simulink model "Assignment1_V6"  (R2022b)
settings: Solver=FixedStepDiscrete  StartTime=0.0  StopTime=10.0  FixedStep=0.001  RelTol=1e-3  EnableMultiTasking=on
undefined symbols (not defined in the file or in its folder): A0, A1, D0, D1, D10, D11, D12, D13, D2, D3, D4, D5, D6, D7, D8, D9, PTA0, PTA1, PTA2, PTB2, PTB23, PTB3, PTB9, PTC16, PTC17, PTC2, PTC3, PTC4, PTD0, PTD1, PTD2, PTD3
libraries: frdmk64flib x19, simulink x4, etargetslib x2
settings Model: ExtModeTrigDuration=5  Creator=a laptop  LastModifiedBy=a laptop
settings SolverCC: AllowMultiTaskInputOutput=on  AutoInsertRateTranBlk=on  InsertRTBMode=Always
settings OptimizationCC: UseSpecifiedMinMax=on  StrengthReduction=on  PassReuseOutputArgsAs=Individual arguments  ZeroExternalMemoryAtStartup=off  ZeroInternalMemoryAtStartup=off  NoFixptDivByZeroProtection=on  EfficientFloat2IntCast=on  MaxStackSize=128  OptimizeBlockOrder=speed  OptimizationPriority=Speed  OptimizationCustomize=off  MultiThreadedLoops=on  EfficientTunableParamExpr=on
settings DebuggingCC: ParameterTunabilityLossMsg=error
settings HardwareCC: ProdBitPerPointer=32  ProdBitPerSizeT=32  ProdBitPerPtrDiffT=32  ProdLargestAtomicInteger=Long  ProdLargestAtomicFloat=Double  ProdWordSize=32  ProdLongLongMode=on  ProdHWDeviceType=ARM Compatible->ARM Cortex
settings SFSimCC: MATLABDynamicMemAlloc=off
settings RTWCC: Description=Embedded Coder  SystemTargetFile=ert.tlc  HardwareBoard=NXP FRDM-K64F  TLCOptions="-aInlineSetEventsForThisBaseRateFcn=TLC_FALSE -aSuppressMultiTaskScheduler=TLC_FALSE  -aRateBasedStepFcn=0"  TemplateMakefile=ert_default_tmf  Toolchain=GNU Tools for ARM Embedded Processors  BuildConfiguration=Faster Runs
settings CodeAppCC: ForceParamTrailComments=on  IgnoreCustomStorageClasses=off  OperatorAnnotations=on  SimulinkDataObjDesc=on  SFDataObjDesc=on  InsertBlockDesc=on
settings ERTTargetCC: SupportNonFinite=off  SupportComplex=off  SupportVariableSizeSignals=on  ExtModeTransport=4  ExtModeMexFile=sendToCommService

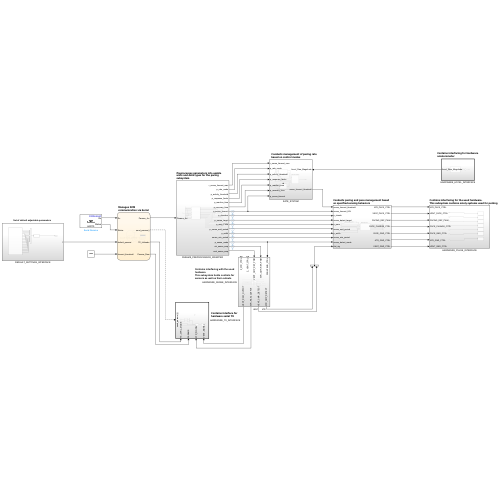
[thumbnail: Simulink's stored preview of the top-level diagram]
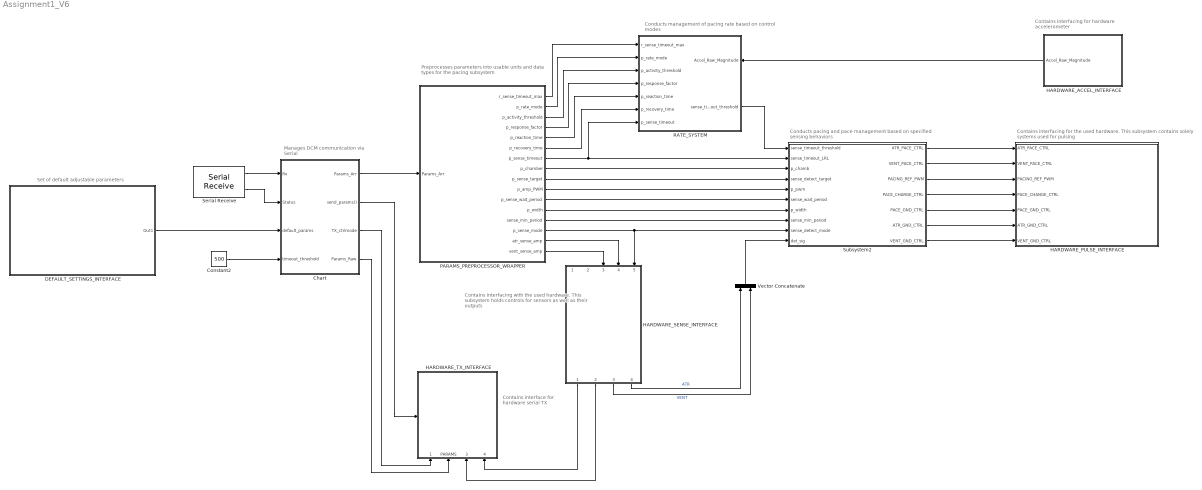
== system Assignment1_V6 ==
  note: Manages DCM communication via Serial
  note: Contains interface for hardware serial TX
  note: Contains interfacing for hardware accelerometer
  note: Conducts management of pacing rate based on control modes
  note: Set of default adjustable parameters
  note: Conducts pacing and pace management based on specified sensing behaviors
  note: Preprocesses parameters into usable units and data types for the pacing subsystem
  note: Contains interfacing for the used hardware.
      | This subsystem contains solely systems used for pulsing
  note: Contains interfacing with the used hardware.
      | This subsystem holds controls for sensors as well as their outputs
  Chart : Stateflow chart  TreatAsAtomicUnit=on
      settings: PortSchema="{\"entries\":[{\"content\":{\"sides\":[{\"content\":{\"connectorIds\":[\"In1\",\"In2\",\"In3\",\"In4\"]},\"type\":\"ConnectorPlacement.EquallySpacedRectSide\",\"uuid\":\"320bc760-8283-4f2b-996b-2bacb632d8d9\"},{\"content\":{\"connectorIds\":[\"Out2\",\"Out4\",\"Out3\",\"Out1\"],\"side\":\"RIGHT\"},\"type\":\"ConnectorPlacement.EquallySpacedRectSide\",\"uuid\":\"405a4bb2-50d6-4c0d-b540-a004b1136e76\"},{\"content\":{\"connectorIds\":[],\"side\":\"TOP\"},\"type\":\"ConnectorPlacement.EquallySpacedRectSide\",\"uuid\":\"abc74140-9996-448b-8aab-969529bb67e5\"}]},\"type\":\"ConnectorPlacement.EquallySpacedConnector\",\"uuid\":\"83b64870-f027-44a6-ac9f-b34b790ab38f\"}],\"packageUris\":[\"http://schema.mathworks.com/mf0/Connector/R2020b\"],\"version\":\"1.0\"}"
  Constant2 : Constant  Value=500
  DEFAULT_SETTINGS_INTERFACE : Subsystem
  HARDWARE_ACCEL_INTERFACE : Subsystem  TreatAsAtomicUnit=on
  HARDWARE_PULSE_INTERFACE : Subsystem
  HARDWARE_SENSE_INTERFACE : Subsystem
  HARDWARE_TX_INTERFACE : Subsystem
  PARAMS_PREPROCESSOR_WRAPPER : Subsystem
  RATE_SYSTEM : Subsystem
      settings: PortSchema="{\"entries\":[{\"content\":{\"sides\":[{\"content\":{\"connectorIds\":[\"In1\",\"In2\",\"In3\",\"In4\",\"In5\",\"In6\",\"In7\"]},\"type\":\"ConnectorPlacement.EquallySpacedRectSide\",\"uuid\":\"da911c89-d0b6-46c9-8ca4-48906cb25f38\"},{\"content\":{\"connectorIds\":[\"In8\",\"Out1\"],\"side\":\"RIGHT\"},\"type\":\"ConnectorPlacement.EquallySpacedRectSide\",\"uuid\":\"d13d5404-7ff7-47d0-a9a2-e0a3ff932734\"},{\"content\":{\"connectorIds\":[],\"side\":\"TOP\"},\"type\":\"ConnectorPlacement.EquallySpacedRectSide\",\"uuid\":\"daee8f81-06de-4c9b-88e4-466b0c826808\"}]},\"type\":\"ConnectorPlacement.EquallySpacedConnector\",\"uuid\":\"a6134fa8-7280-4bb4-a6f1-cb05dfad6031\"}],\"packageUris\":[\"http://schema.mathworks.com/mf0/Connector/R2020b\"],\"version\":\"1.0\"}"
  Serial Receive : frdmk64flib/Serial Receive  SCIModule=0  Baudrate=uint32(9600)  Parity=None  StopBits=1  HardwareFlowControl=None  ByteOrder=LittleEndian  DataType=uint8  DataLength=16  BlockingMode=off  OutputStatus=on  SampleTime=-1
  Subsystem2 : Subsystem
  Vector Concatenate : Concatenate
  wires:
  Serial Receive/1 -> Chart/1(Rx)
  HARDWARE_SENSE_INTERFACE/4(ATR_CMP_DETECT) -> Vector Concatenate/1  "ATR"
  Constant2/1 -> Chart/4(timeout_threshold)
  HARDWARE_SENSE_INTERFACE/3(VENT_CMP_DETECT) -> Vector Concatenate/2  "VENT"
  PARAMS_PREPROCESSOR_WRAPPER/1(r_sense_timeout_max) -> RATE_SYSTEM/1(r_sense_timeout_max)
  HARDWARE_SENSE_INTERFACE/2(ATR_RAW_OUTPUT) -> HARDWARE_TX_INTERFACE/3(ATR_SIGNAL)
  Serial Receive/2 -> Chart/2(Status)
  PARAMS_PREPROCESSOR_WRAPPER/5(p_reaction_time) -> RATE_SYSTEM/5(p_reaction_time)
  Chart/3(TX_ctrlmode) -> HARDWARE_TX_INTERFACE/1(TX_CTRL_MODE)
  PARAMS_PREPROCESSOR_WRAPPER/6(p_recovery_time) -> RATE_SYSTEM/6(p_recovery_time)
  PARAMS_PREPROCESSOR_WRAPPER/14(p_sense_mode) -> Subsystem2/9(sense_detect_mode), HARDWARE_SENSE_INTERFACE/5(FRONTEND_CTRL)
  PARAMS_PREPROCESSOR_WRAPPER/2(p_rate_mode) -> RATE_SYSTEM/2(p_rate_mode)
  PARAMS_PREPROCESSOR_WRAPPER/4(p_response_factor) -> RATE_SYSTEM/4(p_response_factor)
  Chart/1(Params_Raw) -> HARDWARE_TX_INTERFACE/2(PARAMS)
  PARAMS_PREPROCESSOR_WRAPPER/16(vent_sense_amp) -> HARDWARE_SENSE_INTERFACE/3(VENT_CMP_REF_PWM)
  PARAMS_PREPROCESSOR_WRAPPER/3(p_activity_threshold) -> RATE_SYSTEM/3(p_activity_threshold)
  HARDWARE_SENSE_INTERFACE/1(VENT_RAW_OUTPUT) -> HARDWARE_TX_INTERFACE/4(VENT_SIGNAL)
  PARAMS_PREPROCESSOR_WRAPPER/15(atr_sense_amp) -> HARDWARE_SENSE_INTERFACE/4(ATR_CMP_REF_PWM)
  HARDWARE_ACCEL_INTERFACE/1(Accel_Raw_Magnitude) -> RATE_SYSTEM/8(Accel_Raw_Magnitude)
  PARAMS_PREPROCESSOR_WRAPPER/7(p_sense_timeout) -> Subsystem2/2(sense_timeout_LRL), RATE_SYSTEM/7(p_sense_timeout)
  Chart/2(Params_Arr) -> PARAMS_PREPROCESSOR_WRAPPER/1(Params_Arr)
  Chart/4(send_params()) -> HARDWARE_TX_INTERFACE/Trigger
  PARAMS_PREPROCESSOR_WRAPPER/8(p_chamber) -> Subsystem2/3(p_chamb)
  PARAMS_PREPROCESSOR_WRAPPER/9(p_sense_target) -> Subsystem2/4(sense_detect_target)
  RATE_SYSTEM/1(sense_timeout_threshold) -> Subsystem2/1(sense_timeout_threshold)
  PARAMS_PREPROCESSOR_WRAPPER/10(p_amp_PWM) -> Subsystem2/5(p_pwm)
  PARAMS_PREPROCESSOR_WRAPPER/11(p_sense_wait_period) -> Subsystem2/6(sense_wait_period)
  PARAMS_PREPROCESSOR_WRAPPER/12(p_width) -> Subsystem2/7(p_width)
  Vector Concatenate/1 -> Subsystem2/10(det_sig)
  PARAMS_PREPROCESSOR_WRAPPER/13(sense_min_period) -> Subsystem2/8(sense_min_period)
  Subsystem2/1(ATR_PACE_CTRL) -> HARDWARE_PULSE_INTERFACE/1(ATR_PACE_CTRL)
  Subsystem2/2(VENT_PACE_CTRL) -> HARDWARE_PULSE_INTERFACE/2(VENT_PACE_CTRL)
  Subsystem2/3(PACING_REF_PWM) -> HARDWARE_PULSE_INTERFACE/3(PACING_REF_PWM)
  Subsystem2/4(PACE_CHARGE_CTRL) -> HARDWARE_PULSE_INTERFACE/4(PACE_CHANGE_CTRL)
  Subsystem2/5(PACE_GND_CTRL) -> HARDWARE_PULSE_INTERFACE/5(PACE_GND_CTRL)
  Subsystem2/6(ATR_GND_CTRL) -> HARDWARE_PULSE_INTERFACE/6(ATR_GND_CTRL)
  Subsystem2/7(VENT_GND_CTRL) -> HARDWARE_PULSE_INTERFACE/7(VENT_GND_CTRL)
  DEFAULT_SETTINGS_INTERFACE/1(Out1) -> Chart/3(default_params)

== system Assignment1_V6/DEFAULT_SETTINGS_INTERFACE ==
  Cast : DataTypeConversion  OutDataTypeStr=uint8  SaturateOnIntegerOverflow=off  RndMeth=Floor
  DEFAULT_PARAMS : Subsystem
  Vector Concatenate1 : Concatenate  NumInputs=15
  Out1 : Outport
  wires:
  DEFAULT_PARAMS/15(RECOVERY_TIME) -> Vector Concatenate1/15
  DEFAULT_PARAMS/9(VENT_PULSE_WIDTH) -> Vector Concatenate1/9
  DEFAULT_PARAMS/3(UPPER_RATE_LIMIT) -> Vector Concatenate1/3
  Vector Concatenate1/1 -> Cast/1
  DEFAULT_PARAMS/4(MAXIMUM_SENSOR_RATE) -> Vector Concatenate1/4
  DEFAULT_PARAMS/14(RESPONSE_FAC) -> Vector Concatenate1/14
  DEFAULT_PARAMS/7(ATR_SENSE_THRESHOLD) -> Vector Concatenate1/7
  DEFAULT_PARAMS/6(ATR_PULSE_WIDTH) -> Vector Concatenate1/6
  DEFAULT_PARAMS/1(PACE_MODE) -> Vector Concatenate1/1
  DEFAULT_PARAMS/8(VENT_PUL_AMPLITUDE) -> Vector Concatenate1/8
  DEFAULT_PARAMS/12(VENT_REFRACTORY_PERIOD) -> Vector Concatenate1/12
  DEFAULT_PARAMS/10(VENT_SENSE_THRESHOLD) -> Vector Concatenate1/10
  DEFAULT_PARAMS/13(REACTION_TIME) -> Vector Concatenate1/13
  DEFAULT_PARAMS/5(ATR_PUL_AMPLITUDE) -> Vector Concatenate1/5
  DEFAULT_PARAMS/2(LOWER_RATE_LIMIT) -> Vector Concatenate1/2
  DEFAULT_PARAMS/11(ATR_REFRACTORY_PERIOD) -> Vector Concatenate1/11
  Cast/1 -> Out1/1

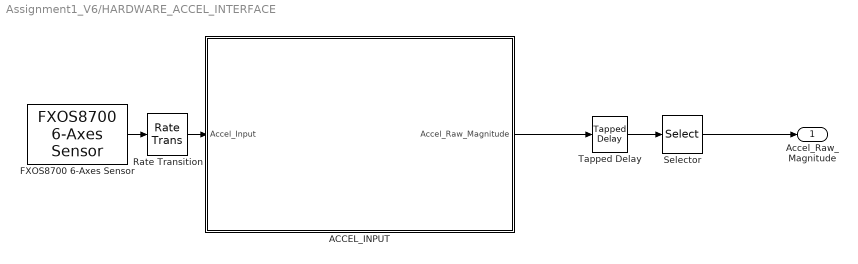
== system Assignment1_V6/HARDWARE_ACCEL_INTERFACE ==
  ACCEL_INPUT : Subsystem
  FXOS8700 6-Axes Sensor : frdmk64flib/FXOS8700 6-Axes Sensor  Activesensor=Accelerometer only  ODR=800Hz  HybridODR=400Hz  Accelfullrange=-4g to +4g  SampleTime=-1
  Rate Transition : RateTransition  Deterministic=off  OutPortSampleTime=0.002
  Selector : Selector  InputPortWidth=50  IndexOptions=Index vector (dialog)  Indices=1  OutputSizes=1
  Tapped Delay : simulink/Discrete/Tapped Delay  vinit=0.0  samptime=0.002  NumDelays=49  DelayOrder=Oldest  includeCurrent=on
  Accel_Raw_Magnitude : Outport
  wires:
  FXOS8700 6-Axes Sensor/1 -> Rate Transition/1
  Tapped Delay/1 -> Selector/1
  Selector/1 -> Accel_Raw_Magnitude/1
  ACCEL_INPUT/1(Accel_Raw_Magnitude) -> Tapped Delay/1
  Rate Transition/1 -> ACCEL_INPUT/1(Accel_Input)

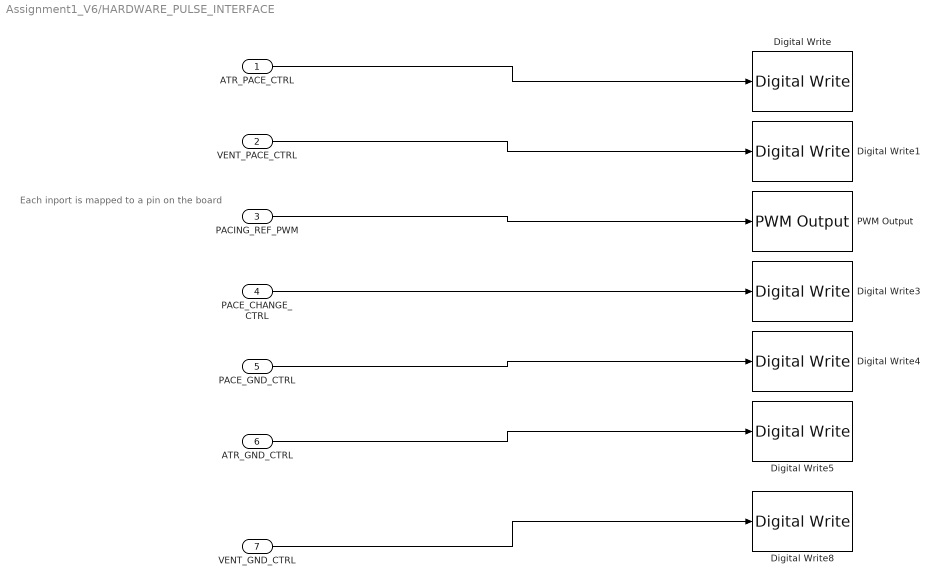
== system Assignment1_V6/HARDWARE_PULSE_INTERFACE ==
  note: Each inport is mapped to a pin on the board
  ATR_PACE_CTRL : Inport
  VENT_PACE_CTRL : Inport  Port=2
  PACING_REF_PWM : Inport  Port=3
  PACE_CHANGE_CTRL : Inport  Port=4
  PACE_GND_CTRL : Inport  Port=5
  ATR_GND_CTRL : Inport  Port=6
  VENT_GND_CTRL : Inport  Port=7
  Digital Write : frdmk64flib/Digital Write  Whichpin=PTA0 (D8)
  Digital Write1 : frdmk64flib/Digital Write  Whichpin=PTC4 (D9)
  Digital Write3 : frdmk64flib/Digital Write  Whichpin=PTB9 (D2)
  Digital Write4 : frdmk64flib/Digital Write  Whichpin=PTD0 (D10)
  Digital Write5 : frdmk64flib/Digital Write  Whichpin=PTD2 (D11)
  Digital Write8 : frdmk64flib/Digital Write  Whichpin=PTD3 (D12)
  PWM Output : frdmk64flib/PWM Output  Whichpin=PTA2 (D5)  InitialFrequency=2000  InitialDutyCycle=0
  wires:
  PACE_CHANGE_CTRL/1 -> Digital Write3/1
  PACE_GND_CTRL/1 -> Digital Write4/1
  VENT_PACE_CTRL/1 -> Digital Write1/1
  VENT_GND_CTRL/1 -> Digital Write8/1
  ATR_PACE_CTRL/1 -> Digital Write/1
  ATR_GND_CTRL/1 -> Digital Write5/1
  PACING_REF_PWM/1 -> PWM Output/1

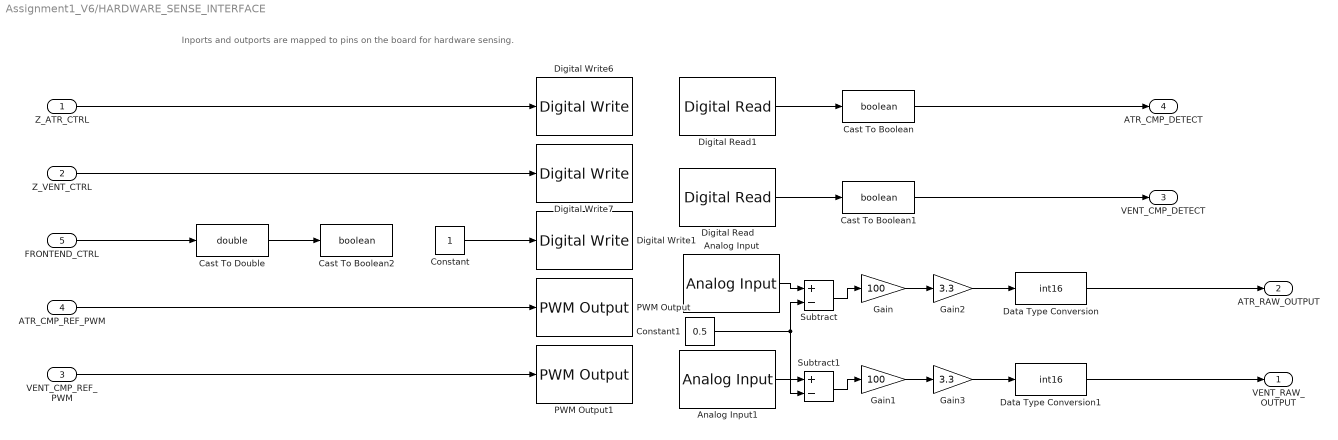
== system Assignment1_V6/HARDWARE_SENSE_INTERFACE ==
  note: Inports and outports are mapped to pins on the board for hardware sensing.
  Z_ATR_CTRL : Inport
  Z_VENT_CTRL : Inport  Port=2
  VENT_CMP_REF_PWM : Inport  Port=3
  ATR_CMP_REF_PWM : Inport  Port=4
  FRONTEND_CTRL : Inport  Port=5
  Analog Input : frdmk64flib/Analog Input  Whichpin=PTB2 (A0)  SampleTime=-1
  Analog Input1 : frdmk64flib/Analog Input  Whichpin=PTB3 (A1)  SampleTime=-1
  Cast To Boolean : DataTypeConversion  OutDataTypeStr=boolean  RndMeth=Round  SaturateOnIntegerOverflow=off
  Cast To Boolean1 : DataTypeConversion  OutDataTypeStr=boolean  RndMeth=Round  SaturateOnIntegerOverflow=off
  Cast To Boolean2 : DataTypeConversion  OutDataTypeStr=boolean  SaturateOnIntegerOverflow=off  RndMeth=Floor
  Cast To Double : DataTypeConversion  OutDataTypeStr=double  SaturateOnIntegerOverflow=off  RndMeth=Floor
  Constant : Constant
  Constant1 : Constant  Value=0.5
  Data Type Conversion : DataTypeConversion  OutDataTypeStr=int16  RndMeth=Nearest  SaturateOnIntegerOverflow=off
  Data Type Conversion1 : DataTypeConversion  OutDataTypeStr=int16  RndMeth=Nearest  SaturateOnIntegerOverflow=off
  Digital Read : frdmk64flib/Digital Read  Whichpin=PTC17 (D1)  SampleTime=-1
  Digital Read1 : frdmk64flib/Digital Read  Whichpin=PTC16 (D0)  SampleTime=-1
  Digital Write1 : frdmk64flib/Digital Write  Whichpin=PTD1 (D13)
  Digital Write6 : frdmk64flib/Digital Write  Whichpin=PTB23 (D4)
  Digital Write7 : frdmk64flib/Digital Write  Whichpin=PTC3 (D7)
  Gain : Gain  Gain=100
  Gain1 : Gain  Gain=100
  Gain2 : Gain  Gain=3.3
  Gain3 : Gain  Gain=3.3
  PWM Output : frdmk64flib/PWM Output  Whichpin=PTC2 (D6)  InitialFrequency=2000  InitialDutyCycle=0
  PWM Output1 : frdmk64flib/PWM Output  Whichpin=PTA1 (D3)  InitialFrequency=2000  InitialDutyCycle=0
  Subtract : Sum  Inputs=+-
  Subtract1 : Sum  Inputs=+-
  VENT_RAW_OUTPUT : Outport
  ATR_RAW_OUTPUT : Outport  Port=2
  VENT_CMP_DETECT : Outport  Port=3
  ATR_CMP_DETECT : Outport  Port=4  OutDataTypeStr=boolean
  wires:
  Z_ATR_CTRL/1 -> Digital Write6/1
  Z_VENT_CTRL/1 -> Digital Write7/1
  FRONTEND_CTRL/1 -> Cast To Double/1
  ATR_CMP_REF_PWM/1 -> PWM Output/1
  VENT_CMP_REF_PWM/1 -> PWM Output1/1
  Digital Read1/1 -> Cast To Boolean/1
  Digital Read/1 -> Cast To Boolean1/1
  Cast To Double/1 -> Cast To Boolean2/1
  Gain/1 -> Gain2/1
  Gain1/1 -> Gain3/1
  Data Type Conversion/1 -> ATR_RAW_OUTPUT/1
  Data Type Conversion1/1 -> VENT_RAW_OUTPUT/1
  Gain2/1 -> Data Type Conversion/1
  Gain3/1 -> Data Type Conversion1/1
  Constant/1 -> Digital Write1/1
  Analog Input/1 -> Subtract/1
  Subtract/1 -> Gain/1
  Analog Input1/1 -> Subtract1/1
  Subtract1/1 -> Gain1/1
  Constant1/1 -> Subtract1/2, Subtract/2
  Cast To Boolean/1 -> ATR_CMP_DETECT/1
  Cast To Boolean1/1 -> VENT_CMP_DETECT/1

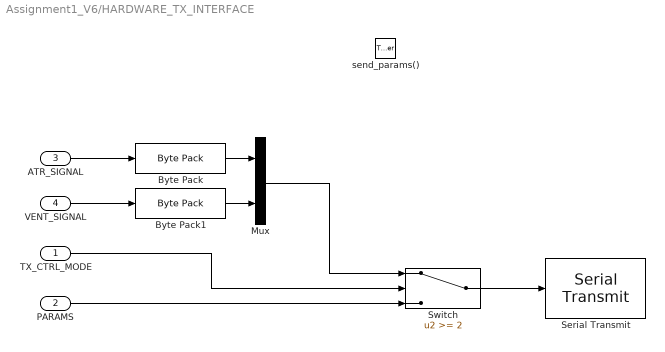
== system Assignment1_V6/HARDWARE_TX_INTERFACE ==
  TX_CTRL_MODE : Inport
  PARAMS : Inport  Port=2  OutDataTypeStr=uint8
  ATR_SIGNAL : Inport  Port=3
  VENT_SIGNAL : Inport  Port=4
  send_params() : TriggerPort  TriggerType=function-call  FunctionName=send_params  VariantControl=(inherit)
  Byte Pack : etargetslib/Byte Pack  datatypes={'int16'}  byteAlign=1
  Byte Pack1 : etargetslib/Byte Pack  datatypes={'int16'}  byteAlign=1
  Mux : Mux  Inputs=2
  Serial Transmit : frdmk64flib/Serial Transmit  SCIModule=0  Baudrate=uint32(9600)  Parity=None  StopBits=1  HardwareFlowControl=None  ByteOrder=LittleEndian  BlockingMode=on  OutputStatus=off
  Switch : Switch  Threshold=2  OutDataTypeStr=uint8  SaturateOnIntegerOverflow=off  InputSameDT=off
  wires:
  Byte Pack1/1 -> Mux/2
  Byte Pack/1 -> Mux/1
  ATR_SIGNAL/1 -> Byte Pack/1
  VENT_SIGNAL/1 -> Byte Pack1/1
  Switch/1 -> Serial Transmit/1
  Mux/1 -> Switch/1
  TX_CTRL_MODE/1 -> Switch/2
  PARAMS/1 -> Switch/3

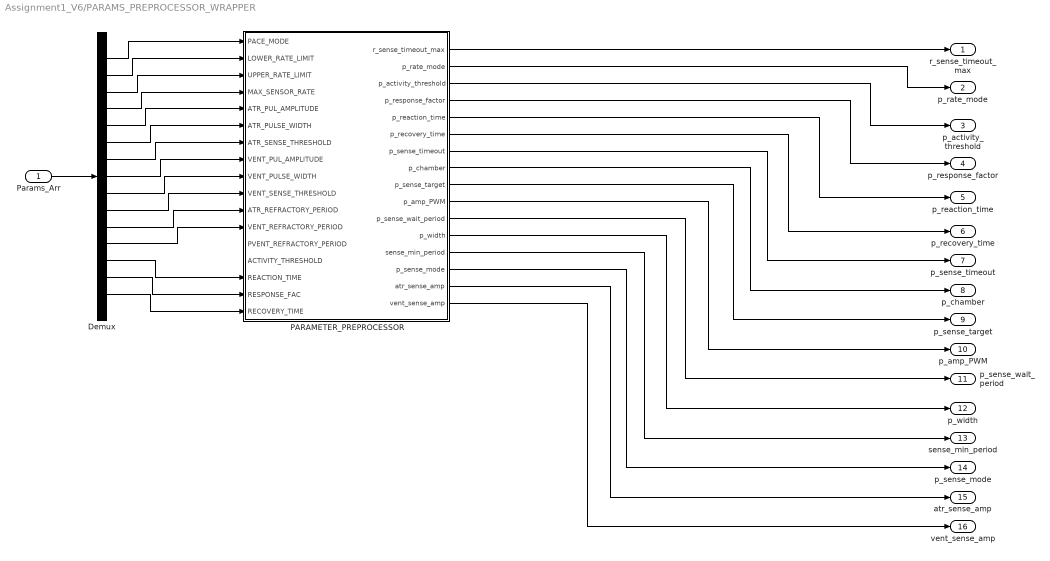
== system Assignment1_V6/PARAMS_PREPROCESSOR_WRAPPER ==
  Params_Arr : Inport
  Demux : Demux  Outputs=15
  PARAMETER_PREPROCESSOR : Subsystem
  r_sense_timeout_max : Outport
  p_rate_mode : Outport  Port=2
  p_activity_threshold : Outport  Port=3
  p_response_factor : Outport  Port=4
  p_reaction_time : Outport  Port=5
  p_recovery_time : Outport  Port=6
  p_sense_timeout : Outport  Port=7
  p_chamber : Outport  Port=8
  p_sense_target : Outport  Port=9
  p_amp_PWM : Outport  Port=10
  p_sense_wait_period : Outport  Port=11
  p_width : Outport  Port=12
  sense_min_period : Outport  Port=13
  p_sense_mode : Outport  Port=14
  atr_sense_amp : Outport  Port=15
  vent_sense_amp : Outport  Port=16
  wires:
  PARAMETER_PREPROCESSOR/11(p_sense_wait_period) -> p_sense_wait_period/1
  PARAMETER_PREPROCESSOR/9(p_sense_target) -> p_sense_target/1
  PARAMETER_PREPROCESSOR/8(p_chamber) -> p_chamber/1
  PARAMETER_PREPROCESSOR/3(p_activity_threshold) -> p_activity_threshold/1
  PARAMETER_PREPROCESSOR/16(vent_sense_amp) -> vent_sense_amp/1
  PARAMETER_PREPROCESSOR/12(p_width) -> p_width/1
  PARAMETER_PREPROCESSOR/15(atr_sense_amp) -> atr_sense_amp/1
  PARAMETER_PREPROCESSOR/14(p_sense_mode) -> p_sense_mode/1
  PARAMETER_PREPROCESSOR/5(p_reaction_time) -> p_reaction_time/1
  PARAMETER_PREPROCESSOR/10(p_amp_PWM) -> p_amp_PWM/1
  PARAMETER_PREPROCESSOR/13(sense_min_period) -> sense_min_period/1
  PARAMETER_PREPROCESSOR/1(r_sense_timeout_max) -> r_sense_timeout_max/1
  PARAMETER_PREPROCESSOR/4(p_response_factor) -> p_response_factor/1
  PARAMETER_PREPROCESSOR/2(p_rate_mode) -> p_rate_mode/1
  PARAMETER_PREPROCESSOR/7(p_sense_timeout) -> p_sense_timeout/1
  PARAMETER_PREPROCESSOR/6(p_recovery_time) -> p_recovery_time/1
  Params_Arr/1 -> Demux/1
  Demux/15 -> PARAMETER_PREPROCESSOR/17(RECOVERY_TIME)
  Demux/14 -> PARAMETER_PREPROCESSOR/16(RESPONSE_FAC)
  Demux/13 -> PARAMETER_PREPROCESSOR/15(REACTION_TIME)
  Demux/12 -> PARAMETER_PREPROCESSOR/12(VENT_REFRACTORY_PERIOD)
  Demux/11 -> PARAMETER_PREPROCESSOR/11(ATR_REFRACTORY_PERIOD)
  Demux/10 -> PARAMETER_PREPROCESSOR/10(VENT_SENSE_THRESHOLD)
  Demux/9 -> PARAMETER_PREPROCESSOR/9(VENT_PULSE_WIDTH)
  Demux/8 -> PARAMETER_PREPROCESSOR/8(VENT_PUL_AMPLITUDE)
  Demux/7 -> PARAMETER_PREPROCESSOR/7(ATR_SENSE_THRESHOLD)
  Demux/6 -> PARAMETER_PREPROCESSOR/6(ATR_PULSE_WIDTH)
  Demux/5 -> PARAMETER_PREPROCESSOR/5(ATR_PUL_AMPLITUDE)
  Demux/4 -> PARAMETER_PREPROCESSOR/4(MAX_SENSOR_RATE)
  Demux/3 -> PARAMETER_PREPROCESSOR/3(UPPER_RATE_LIMIT)
  Demux/2 -> PARAMETER_PREPROCESSOR/2(LOWER_RATE_LIMIT)
  Demux/1 -> PARAMETER_PREPROCESSOR/1(PACE_MODE)

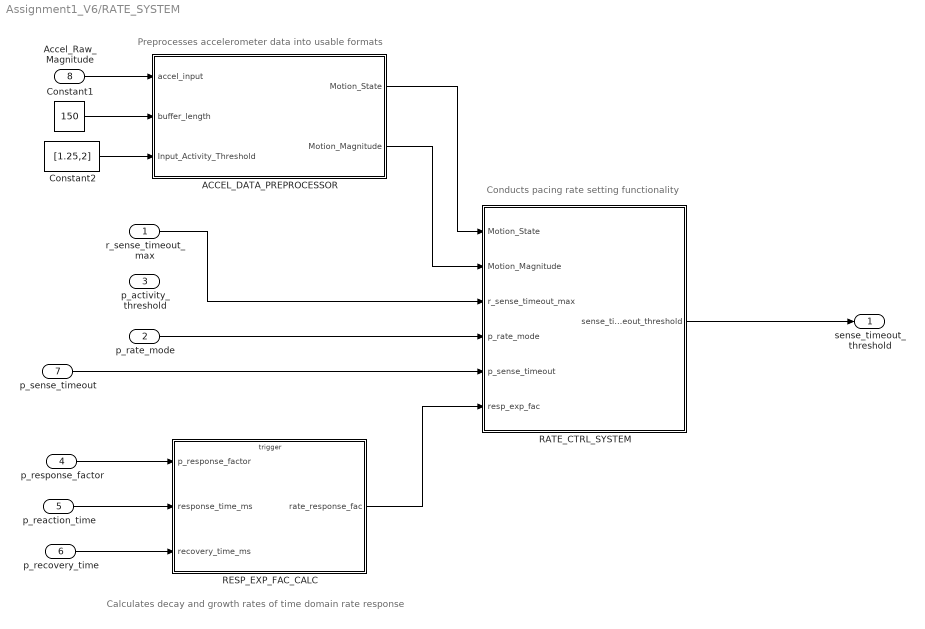
== system Assignment1_V6/RATE_SYSTEM ==
  note: Preprocesses accelerometer data into usable formats
  note: Calculates decay and growth rates of time domain rate response
  note: Conducts pacing rate setting functionality
  r_sense_timeout_max : Inport
  p_rate_mode : Inport  Port=2
  p_activity_threshold : Inport  Port=3
  p_response_factor : Inport  Port=4
  p_reaction_time : Inport  Port=5
  p_recovery_time : Inport  Port=6
  p_sense_timeout : Inport  Port=7
  Accel_Raw_Magnitude : Inport  Port=8
  ACCEL_DATA_PREPROCESSOR : Subsystem
  Constant1 : Constant  Value=150
  Constant2 : Constant  Value=[1.25,2]
  RATE_CTRL_SYSTEM : Stateflow chart  TreatAsAtomicUnit=on
  RESP_EXP_FAC_CALC : Subsystem
  sense_timeout_threshold : Outport
  wires:
  p_rate_mode/1 -> RATE_CTRL_SYSTEM/4(p_rate_mode)
  r_sense_timeout_max/1 -> RATE_CTRL_SYSTEM/3(r_sense_timeout_max)
  p_sense_timeout/1 -> RATE_CTRL_SYSTEM/5(p_sense_timeout)
  Constant2/1 -> ACCEL_DATA_PREPROCESSOR/3(Input_Activity_Threshold)
  Constant1/1 -> ACCEL_DATA_PREPROCESSOR/2(buffer_length)
  Accel_Raw_Magnitude/1 -> ACCEL_DATA_PREPROCESSOR/1(accel_input)
  RATE_CTRL_SYSTEM/1(sense_timeout_threshold) -> sense_timeout_threshold/1
  ACCEL_DATA_PREPROCESSOR/2(Motion_Magnitude) -> RATE_CTRL_SYSTEM/2(Motion_Magnitude)
  ACCEL_DATA_PREPROCESSOR/1(Motion_State) -> RATE_CTRL_SYSTEM/1(Motion_State)
  p_response_factor/1 -> RESP_EXP_FAC_CALC/1(p_response_factor)
  p_reaction_time/1 -> RESP_EXP_FAC_CALC/2(response_time_ms)
  p_recovery_time/1 -> RESP_EXP_FAC_CALC/3(recovery_time_ms)
  RESP_EXP_FAC_CALC/1(rate_response_fac) -> RATE_CTRL_SYSTEM/6(resp_exp_fac)

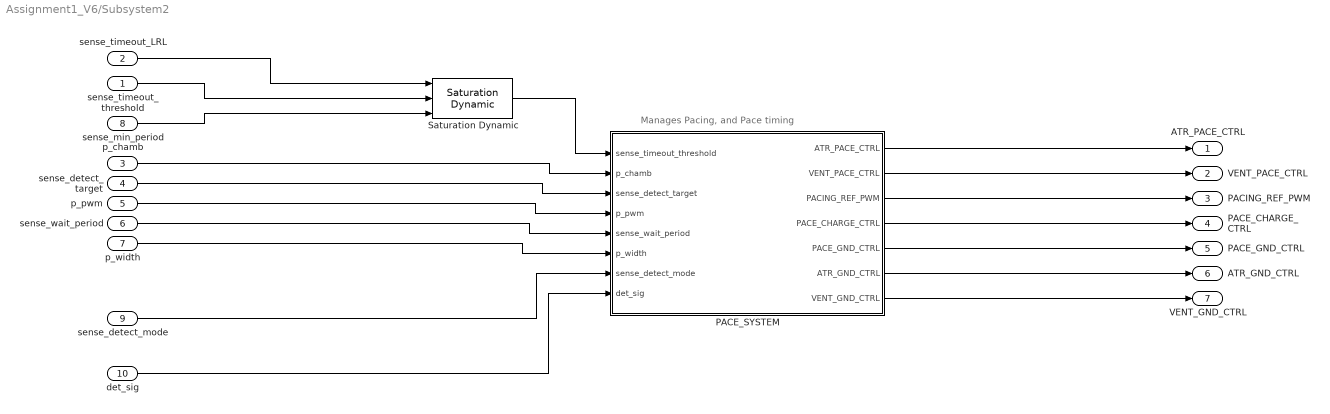
== system Assignment1_V6/Subsystem2 ==
  note: Manages Pacing, and Pace timing
  sense_timeout_threshold : Inport
  sense_timeout_LRL : Inport  Port=2
  p_chamb : Inport  Port=3
  sense_detect_target : Inport  Port=4
  p_pwm : Inport  Port=5
  sense_wait_period : Inport  Port=6
  p_width : Inport  Port=7
  sense_min_period : Inport  Port=8
  sense_detect_mode : Inport  Port=9
  det_sig : Inport  Port=10
  PACE_SYSTEM : Stateflow chart  TreatAsAtomicUnit=on
      settings: PortSchema="{\"entries\":[{\"content\":{\"sides\":[{\"content\":{\"connectorIds\":[\"In3\",\"In1\",\"In2\",\"In4\",\"In5\",\"In6\",\"In7\",\"In8\"]},\"type\":\"ConnectorPlacement.EquallySpacedRectSide\",\"uuid\":\"7443a3c3-e653-4ca7-8541-eabcfaf454bc\"},{\"content\":{\"connectorIds\":[\"Out1\",\"Out2\",\"Out3\",\"Out4\",\"Out5\",\"Out6\",\"Out7\"],\"side\":\"RIGHT\"},\"type\":\"ConnectorPlacement.EquallySpacedRectSide\",\"uuid\":\"2c63cfa0-dfd9-4a62-91aa-a60ecd75cc2c\"},{\"content\":{\"connectorIds\":[],\"side\":\"TOP\"},\"type\":\"ConnectorPlacement.EquallySpacedRectSide\",\"uuid\":\"5c2dbe0e-7e89-449d-bdd0-c0f7e700edae\"}]},\"type\":\"ConnectorPlacement.EquallySpacedConnector\",\"uuid\":\"602c7a1c-8730-4b31-b945-266bd0371e8b\"}],\"packageUris\":[\"http://schema.mathworks.com/mf0/Connector/R2020b\"],\"version\":\"1.0\"}"
  Saturation Dynamic : simulink/Discontinuities/Saturation Dynamic  OutMin=[]  OutMax=[]  OutDataTypeStr=Inherit: Same as second input  OutDataType=fixdt(1, 16)  OutScaling=2^-10  DoSatur=off
  ATR_PACE_CTRL : Outport
  VENT_PACE_CTRL : Outport  Port=2
  PACING_REF_PWM : Outport  Port=3
  PACE_CHARGE_CTRL : Outport  Port=4
  PACE_GND_CTRL : Outport  Port=5
  ATR_GND_CTRL : Outport  Port=6
  VENT_GND_CTRL : Outport  Port=7
  wires:
  PACE_SYSTEM/3(PACING_REF_PWM) -> PACING_REF_PWM/1
  p_pwm/1 -> PACE_SYSTEM/4(p_pwm)
  p_chamb/1 -> PACE_SYSTEM/1(p_chamb)
  sense_detect_target/1 -> PACE_SYSTEM/2(sense_detect_target)
  sense_wait_period/1 -> PACE_SYSTEM/5(sense_wait_period)
  PACE_SYSTEM/7(VENT_GND_CTRL) -> VENT_GND_CTRL/1
  sense_detect_mode/1 -> PACE_SYSTEM/7(sense_detect_mode)
  PACE_SYSTEM/5(PACE_GND_CTRL) -> PACE_GND_CTRL/1
  PACE_SYSTEM/1(ATR_PACE_CTRL) -> ATR_PACE_CTRL/1
  PACE_SYSTEM/2(VENT_PACE_CTRL) -> VENT_PACE_CTRL/1
  det_sig/1 -> PACE_SYSTEM/8(det_sig)
  p_width/1 -> PACE_SYSTEM/6(p_width)
  PACE_SYSTEM/6(ATR_GND_CTRL) -> ATR_GND_CTRL/1
  PACE_SYSTEM/4(PACE_CHARGE_CTRL) -> PACE_CHARGE_CTRL/1
  sense_timeout_threshold/1 -> Saturation Dynamic/2
  sense_timeout_LRL/1 -> Saturation Dynamic/1
  sense_min_period/1 -> Saturation Dynamic/3
  Saturation Dynamic/1 -> PACE_SYSTEM/3(sense_timeout_threshold)

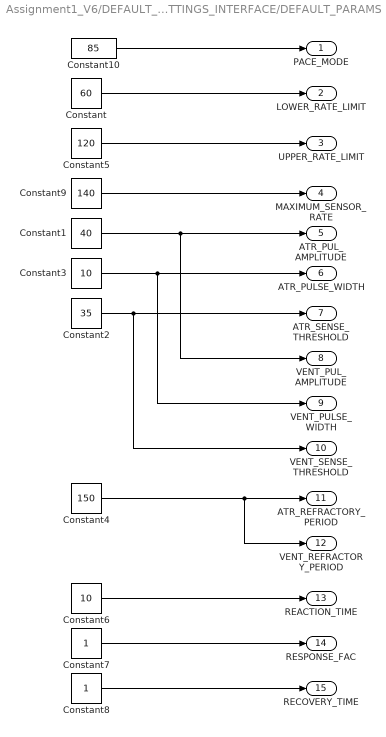
== system Assignment1_V6/DEFAULT_SETTINGS_INTERFACE/DEFAULT_PARAMS ==
  Constant : Constant  Value=60
  Constant1 : Constant  Value=40
  Constant10 : Constant  Value=85
  Constant2 : Constant  Value=35
  Constant3 : Constant  Value=10
  Constant4 : Constant  Value=150
  Constant5 : Constant  Value=120
  Constant6 : Constant  Value=10
  Constant7 : Constant
  Constant8 : Constant
  Constant9 : Constant  Value=140
  PACE_MODE : Outport
  LOWER_RATE_LIMIT : Outport  Port=2
  UPPER_RATE_LIMIT : Outport  Port=3
  MAXIMUM_SENSOR_RATE : Outport  Port=4
  ATR_PUL_AMPLITUDE : Outport  Port=5
  ATR_PULSE_WIDTH : Outport  Port=6
  ATR_SENSE_THRESHOLD : Outport  Port=7
  VENT_PUL_AMPLITUDE : Outport  Port=8
  VENT_PULSE_WIDTH : Outport  Port=9
  VENT_SENSE_THRESHOLD : Outport  Port=10
  ATR_REFRACTORY_PERIOD : Outport  Port=11
  VENT_REFRACTORY_PERIOD : Outport  Port=12
  REACTION_TIME : Outport  Port=13
  RESPONSE_FAC : Outport  Port=14
  RECOVERY_TIME : Outport  Port=15
  wires:
  Constant10/1 -> PACE_MODE/1
  Constant/1 -> LOWER_RATE_LIMIT/1
  Constant1/1 -> VENT_PUL_AMPLITUDE/1, ATR_PUL_AMPLITUDE/1
  Constant2/1 -> ATR_SENSE_THRESHOLD/1, VENT_SENSE_THRESHOLD/1
  Constant3/1 -> ATR_PULSE_WIDTH/1, VENT_PULSE_WIDTH/1
  Constant4/1 -> VENT_REFRACTORY_PERIOD/1, ATR_REFRACTORY_PERIOD/1
  Constant5/1 -> UPPER_RATE_LIMIT/1
  Constant6/1 -> REACTION_TIME/1
  Constant7/1 -> RESPONSE_FAC/1
  Constant8/1 -> RECOVERY_TIME/1
  Constant9/1 -> MAXIMUM_SENSOR_RATE/1

== system Assignment1_V6/HARDWARE_ACCEL_INTERFACE/ACCEL_INPUT ==
  Accel_Input : Inport
  Demux : Demux  Commented=on  Outputs=3
  Dot Product : DotProduct  RndMeth=Nearest  OutDataTypeStr=Inherit: Inherit via internal rule
  MATLAB Function : MATLAB Function  Commented=on  TreatAsAtomicUnit=on
  Square Root : Sqrt
  Accel_Raw_Magnitude : Outport  OutDataTypeStr=double
  wires:
  MATLAB Function/1(Accel_Raw_Magnitude) -> ?
  Dot Product/1 -> Square Root/1
  Accel_Input/1 -> Dot Product/2, Dot Product/1, MATLAB Function/1(Accel_Vector), Demux/1
  Square Root/1 -> Accel_Raw_Magnitude/1

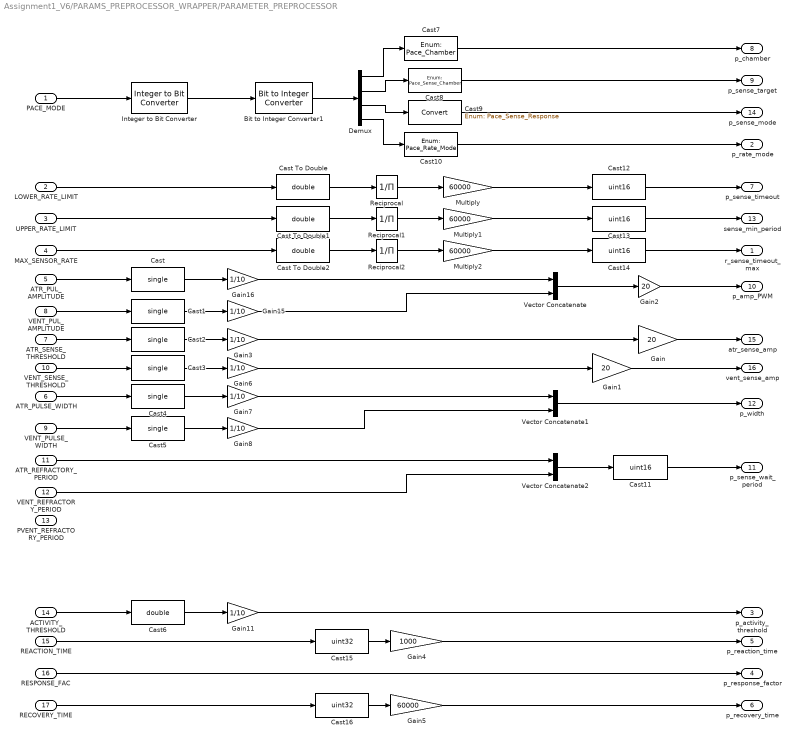
== system Assignment1_V6/PARAMS_PREPROCESSOR_WRAPPER/PARAMETER_PREPROCESSOR ==
  PACE_MODE : Inport
  LOWER_RATE_LIMIT : Inport  Port=2
  UPPER_RATE_LIMIT : Inport  Port=3
  MAX_SENSOR_RATE : Inport  Port=4
  ATR_PUL_AMPLITUDE : Inport  Port=5
  ATR_PULSE_WIDTH : Inport  Port=6
  ATR_SENSE_THRESHOLD : Inport  Port=7
  VENT_PUL_AMPLITUDE : Inport  Port=8
  VENT_PULSE_WIDTH : Inport  Port=9
  VENT_SENSE_THRESHOLD : Inport  Port=10
  ATR_REFRACTORY_PERIOD : Inport  Port=11
  VENT_REFRACTORY_PERIOD : Inport  Port=12
  PVENT_REFRACTORY_PERIOD : Inport  Port=13
  ACTIVITY_THRESHOLD : Inport  Port=14
  REACTION_TIME : Inport  Port=15
  RESPONSE_FAC : Inport  Port=16
  RECOVERY_TIME : Inport  Port=17
  Bit to Integer Converter1 : simulink/Logic and Bit Operations/Bit to Integer Converter  nbits=2  bitOrder=MSB first  signedOutputValues=Unsigned  outDtype=uint8  outDtypeSigned=Inherit via internal rule
  Cast{,1..5} (6 alike) : DataTypeConversion  OutDataTypeStr=single  SaturateOnIntegerOverflow=off  RndMeth=Floor
  Cast To Double : DataTypeConversion  OutDataTypeStr=double  SaturateOnIntegerOverflow=off  RndMeth=Floor
  Cast To Double1 : DataTypeConversion  OutDataTypeStr=double  SaturateOnIntegerOverflow=off  RndMeth=Floor
  Cast To Double2 : DataTypeConversion  OutDataTypeStr=double  SaturateOnIntegerOverflow=off  RndMeth=Floor
  Cast10 : DataTypeConversion  OutDataTypeStr=Enum: Pace_Rate_Mode  SaturateOnIntegerOverflow=off  RndMeth=Floor
  Cast11 : DataTypeConversion  OutDataTypeStr=uint16  SaturateOnIntegerOverflow=off  RndMeth=Floor
  Cast12 : DataTypeConversion  OutDataTypeStr=uint16  SaturateOnIntegerOverflow=off
  Cast13 : DataTypeConversion  OutDataTypeStr=uint16  SaturateOnIntegerOverflow=off  RndMeth=Floor
  Cast14 : DataTypeConversion  OutDataTypeStr=uint16  SaturateOnIntegerOverflow=off
  Cast15 : DataTypeConversion  OutDataTypeStr=uint32  SaturateOnIntegerOverflow=off  RndMeth=Floor
  Cast16 : DataTypeConversion  OutDataTypeStr=uint32  SaturateOnIntegerOverflow=off  RndMeth=Floor
  Cast6 : DataTypeConversion  OutDataTypeStr=double  SaturateOnIntegerOverflow=off  RndMeth=Floor
  Cast7 : DataTypeConversion  OutDataTypeStr=Enum: Pace_Chamber  SaturateOnIntegerOverflow=off  RndMeth=Floor
  Cast8 : DataTypeConversion  OutDataTypeStr=Enum: Pace_Sense_Chamber  SaturateOnIntegerOverflow=off  RndMeth=Floor
  Cast9 : DataTypeConversion  OutDataTypeStr=Enum: Pace_Sense_Response  SaturateOnIntegerOverflow=off  RndMeth=Floor
  Demux : Demux
  Gain : Gain  Gain=20
  Gain1 : Gain  Gain=20
  Gain{3,6..8,11,15..16} (7 alike) : Gain  Gain=1/10
  Gain2 : Gain  Gain=20
  Gain4 : Gain  Gain=1000  OutDataTypeStr=uint32  ParamDataTypeStr=Inherit: Same as input
  Gain5 : Gain  Gain=60000  ParamDataTypeStr=uint32
  Integer to Bit Converter : simulink/Logic and Bit Operations/Integer to Bit Converter  nbits=8  signedInputValues=Unsigned  bitOrder=MSB first  outDtype=uint8
  Multiply : Gain  Gain=60000
  Multiply1 : Gain  Gain=60000
  Multiply2 : Gain  Gain=60000
  Reciprocal : Product  Inputs=/
  Reciprocal1 : Product  Inputs=/
  Reciprocal2 : Product  Inputs=/
  Vector Concatenate : Concatenate
  Vector Concatenate1 : Concatenate
  Vector Concatenate2 : Concatenate
  r_sense_timeout_max : Outport
  p_rate_mode : Outport  Port=2
  p_activity_threshold : Outport  Port=3
  p_response_factor : Outport  Port=4
  p_reaction_time : Outport  Port=5
  p_recovery_time : Outport  Port=6
  p_sense_timeout : Outport  Port=7
  p_chamber : Outport  Port=8
  p_sense_target : Outport  Port=9
  p_amp_PWM : Outport  Port=10
  p_sense_wait_period : Outport  Port=11
  p_width : Outport  Port=12
  sense_min_period : Outport  Port=13
  p_sense_mode : Outport  Port=14
  atr_sense_amp : Outport  Port=15
  vent_sense_amp : Outport  Port=16
  wires:
  Cast8/1 -> p_sense_target/1
  Cast9/1 -> p_sense_mode/1
  ATR_PUL_AMPLITUDE/1 -> Cast/1
  VENT_PUL_AMPLITUDE/1 -> Cast1/1
  Cast7/1 -> p_chamber/1
  ATR_SENSE_THRESHOLD/1 -> Cast2/1
  VENT_SENSE_THRESHOLD/1 -> Cast3/1
  Gain2/1 -> p_amp_PWM/1
  Vector Concatenate/1 -> Gain2/1
  ATR_PULSE_WIDTH/1 -> Cast4/1
  VENT_PULSE_WIDTH/1 -> Cast5/1
  Vector Concatenate1/1 -> p_width/1
  Vector Concatenate2/1 -> Cast11/1
  Cast To Double/1 -> Reciprocal/1
  Multiply/1 -> Cast12/1
  Gain1/1 -> vent_sense_amp/1
  Gain/1 -> atr_sense_amp/1
  Cast10/1 -> p_rate_mode/1
  ACTIVITY_THRESHOLD/1 -> Cast6/1
  Multiply1/1 -> Cast13/1
  Cast To Double1/1 -> Reciprocal1/1
  Multiply2/1 -> Cast14/1
  Cast To Double2/1 -> Reciprocal2/1
  Gain4/1 -> p_reaction_time/1
  Gain5/1 -> p_recovery_time/1
  Reciprocal/1 -> Multiply/1
  Reciprocal1/1 -> Multiply1/1
  Reciprocal2/1 -> Multiply2/1
  PACE_MODE/1 -> Integer to Bit Converter/1
  Gain3/1 -> Gain/1
  Gain6/1 -> Gain1/1
  Gain7/1 -> Vector Concatenate1/1
  Gain8/1 -> Vector Concatenate1/2
  ATR_REFRACTORY_PERIOD/1 -> Vector Concatenate2/1
  VENT_REFRACTORY_PERIOD/1 -> Vector Concatenate2/2
  Gain11/1 -> p_activity_threshold/1
  REACTION_TIME/1 -> Cast15/1
  RESPONSE_FAC/1 -> p_response_factor/1
  RECOVERY_TIME/1 -> Cast16/1
  Gain15/1 -> Vector Concatenate/2
  Gain16/1 -> Vector Concatenate/1
  MAX_SENSOR_RATE/1 -> Cast To Double2/1
  UPPER_RATE_LIMIT/1 -> Cast To Double1/1
  LOWER_RATE_LIMIT/1 -> Cast To Double/1
  Cast/1 -> Gain16/1
  Cast1/1 -> Gain15/1
  Cast2/1 -> Gain3/1
  Cast3/1 -> Gain6/1
  Cast4/1 -> Gain7/1
  Cast5/1 -> Gain8/1
  Cast6/1 -> Gain11/1
  Integer to Bit Converter/1 -> Bit to Integer Converter1/1
  Bit to Integer Converter1/1 -> Demux/1
  Demux/1 -> Cast7/1
  Demux/2 -> Cast8/1
  Demux/3 -> Cast9/1
  Demux/4 -> Cast10/1
  Cast11/1 -> p_sense_wait_period/1
  Cast12/1 -> p_sense_timeout/1
  Cast13/1 -> sense_min_period/1
  Cast14/1 -> r_sense_timeout_max/1
  Cast15/1 -> Gain4/1
  Cast16/1 -> Gain5/1

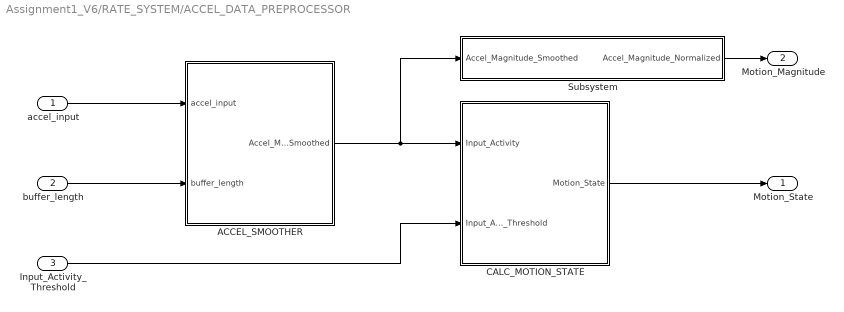
== system Assignment1_V6/RATE_SYSTEM/ACCEL_DATA_PREPROCESSOR ==
  accel_input : Inport
  buffer_length : Inport  Port=2
  Input_Activity_Threshold : Inport  Port=3
  ACCEL_SMOOTHER : Subsystem
  CALC_MOTION_STATE : Subsystem
  Subsystem : Subsystem
  Motion_State : Outport
  Motion_Magnitude : Outport  Port=2
  wires:
  ACCEL_SMOOTHER/1(Accel_Magnitude_Smoothed) -> Subsystem/1(Accel_Magnitude_Smoothed), CALC_MOTION_STATE/1(Input_Activity)
  accel_input/1 -> ACCEL_SMOOTHER/1(accel_input)
  buffer_length/1 -> ACCEL_SMOOTHER/2(buffer_length)
  CALC_MOTION_STATE/1(Motion_State) -> Motion_State/1
  Input_Activity_Threshold/1 -> CALC_MOTION_STATE/2(Input_Activity_Threshold)
  Subsystem/1(Accel_Magnitude_Normalized) -> Motion_Magnitude/1

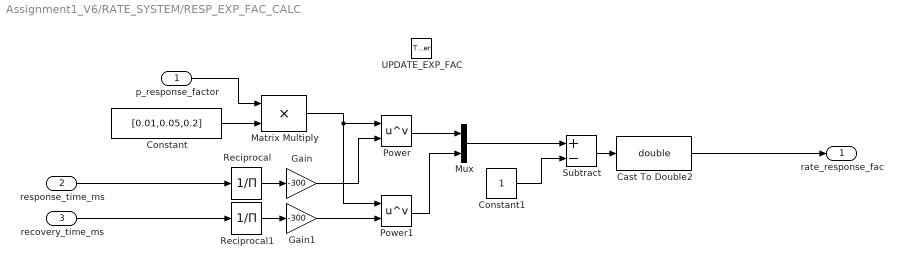
== system Assignment1_V6/RATE_SYSTEM/RESP_EXP_FAC_CALC ==
  p_response_factor : Inport
  response_time_ms : Inport  Port=2
  recovery_time_ms : Inport  Port=3
  UPDATE_EXP_FAC : TriggerPort  TriggerType=function-call  IsSimulinkFunction=on  FunctionName=UPDATE_EXP_FAC  FunctionVisibility=scoped  ScopeName=PORT  VariantControl=(inherit)
  Cast To Double2 : DataTypeConversion  OutDataTypeStr=double  SaturateOnIntegerOverflow=off  RndMeth=Floor
  Constant : Constant  Value=[0.01,0.05,0.2]
  Constant1 : Constant
  Gain : Gain  Gain=-300
  Gain1 : Gain  Gain=-300
  Matrix Multiply : Product
  Mux : Mux  Inputs=2
  Power : Math  Operator=pow
  Power1 : Math  Operator=pow
  Reciprocal : Product  Inputs=/  OutDataTypeStr=double
  Reciprocal1 : Product  Inputs=/  OutDataTypeStr=double
  Subtract : Sum  Inputs=+-
  rate_response_fac : Outport
  wires:
  response_time_ms/1 -> Reciprocal/1
  Matrix Multiply/1 -> Power1/1, Power/1
  Power/1 -> Mux/1
  Subtract/1 -> Cast To Double2/1
  Constant1/1 -> Subtract/2
  Reciprocal/1 -> Gain/1
  Gain/1 -> Power/2
  Power1/1 -> Mux/2
  Mux/1 -> Subtract/1
  Reciprocal1/1 -> Gain1/1
  Gain1/1 -> Power1/2
  Constant/1 -> Matrix Multiply/2
  p_response_factor/1 -> Matrix Multiply/1
  recovery_time_ms/1 -> Reciprocal1/1
  Cast To Double2/1 -> rate_response_fac/1

== system Assignment1_V6/RATE_SYSTEM/ACCEL_DATA_PREPROCESSOR/ACCEL_SMOOTHER ==
  accel_input : Inport
  buffer_length : Inport  Port=2
  Buffer Smooth : Subsystem  Commented=on
  MATLAB Function2 : MATLAB Function  TreatAsAtomicUnit=on
  Accel_Magnitude_Smoothed : Outport
  wires:
  accel_input/1 -> MATLAB Function2/1(input), Buffer Smooth/1(input_data)
  buffer_length/1 -> MATLAB Function2/2(buffer_length), Buffer Smooth/2(buffer_length)
  MATLAB Function2/1(smoothed_output) -> Accel_Magnitude_Smoothed/1

== system Assignment1_V6/RATE_SYSTEM/ACCEL_DATA_PREPROCESSOR/CALC_MOTION_STATE ==
  Input_Activity : Inport
  Input_Activity_Threshold : Inport  Port=2
  MATLAB Function : MATLAB Function  TreatAsAtomicUnit=on
  Motion_State : Outport
  wires:
  Input_Activity/1 -> MATLAB Function/1(Input_Activity)
  Input_Activity_Threshold/1 -> MATLAB Function/2(Input_Activity_Threshold)
  MATLAB Function/1(Motion_State) -> Motion_State/1

== system Assignment1_V6/RATE_SYSTEM/ACCEL_DATA_PREPROCESSOR/Subsystem ==
  Accel_Magnitude_Smoothed : Inport
  Gain : Gain  Gain=30
  Accel_Magnitude_Normalized : Outport
  wires:
  Accel_Magnitude_Smoothed/1 -> Gain/1
  Gain/1 -> Accel_Magnitude_Normalized/1

== system Assignment1_V6/RATE_SYSTEM/ACCEL_DATA_PREPROCESSOR/ACCEL_SMOOTHER/Buffer Smooth ==
  input_data : Inport
  buffer_length : Inport  Port=2  OutMin=1  OutMax=1000
  MATLAB Function : MATLAB Function  TreatAsAtomicUnit=on
  MATLAB Function1 : MATLAB Function  TreatAsAtomicUnit=on
  Smoothed_Output : Outport
  wires:
  input_data/1 -> MATLAB Function/1(input_data)
  MATLAB Function1/1(Smoothed_Output) -> Smoothed_Output/1
  buffer_length/1 -> MATLAB Function1/2(buffer_length), MATLAB Function/2(buffer_length)
  MATLAB Function/1(Buffer_Output) -> MATLAB Function1/1(input_buffer)

== matlab function Assignment1_V6/HARDWARE_ACCEL_INTERFACE/ACCEL_INPUT/MATLAB Function ==
  data: Accel_Vector input; Accel_Raw_Magnitude output
function Accel_Raw_Magnitude = Get_Magnitude(Accel_Vector)
    Accel_Raw_Magnitude = (Accel_Vector(1)^2 + Accel_Vector(2)^2 + Accel_Vector(3)^2)^(1/2);
end

== stateflow chart Assignment1_V6/Subsystem2/PACE_SYSTEM ==
  note: PACE sends pulses to the specified body part
  state PACE
    state Charge
      %Stop discharge of C22
      PACE_GND_CTRL = true;
      VENT_PACE_CTRL = false;
      ATR_PACE_CTRL = false;
      %Discharge blocking capacitor
      if p_chamb == Pace_Chamber.Atrium
      ATR_GND_CTRL = true;
      VENT_GND_CTRL = false;
      else
      ATR_GND_CTRL = false;
      VENT_GND_CTRL = true;
      end
      %Charge C22
      ATR_PACE_CTRL = false;
      VENT_PACE_CTRL = false;
      PACING_REF_PWM = p_pwm(double(p_chamb));
      PACE_CHARGE_CTRL = true;
      send(pace_compl)
    state Discharge_Prep
      %Prepares discharge
      %Stop charging C22
      PACING_REF_PWM = 0;
      PACE_CHARGE_CTRL = false;
      PACE_GND_CTRL = true;
      %Stop discharging blocking capacitor
      ATR_GND_CTRL = false;
      VENT_GND_CTRL = false;
    state Pace_Atr
      ATR_PACE_CTRL = true;
    state Pace_Vent
      VENT_PACE_CTRL = true;
    (default) -> Discharge_Prep
    Pace_Atr -> Charge : after(p_width(double(p_chamb)), msec)
    Discharge_Prep -> Pace_Atr [order 1] : [p_chamb == Pace_Chamber.Atrium]
    Discharge_Prep -> Pace_Vent [order 2] : [p_chamb == Pace_Chamber.Ventricle]
    Pace_Vent -> Charge : after(p_width(double(p_chamb)), msec)
  state SENSE
    state Sense_Finish
    state Sense_Disabled
      %All sensor timing is disabled
    state Sense_Wait
      %Sensor prep
    note: Warm-up period before sensor is active
    state Sense_Detect
      %Sensor active period
    state Sense_Fail
      %disp("HELLO");
      %Starts the pacing process
      send(sense_timeout);
    state Sense_Detected
    note: This state is present for future DCM interactions and data logging
    (default) -> Sense_Finish
    Sense_Finish -> Sense_Disabled [order 2] : [sense_detect_mode == Pace_Sense_Response.Nothing]
    Sense_Finish -> Sense_Wait [order 1] : [sense_detect_mode ~= Pace_Sense_Response.Nothing]
    Sense_Disabled -> Sense_Fail : after(sense_timeout_threshold, msec)
    Sense_Wait -> Sense_Fail [order 1] : [sense_detect_mode == Pace_Sense_Response.Nothing]
    Sense_Detected -> Sense_Wait
    Sense_Wait -> Sense_Detect [order 2] : after(sense_wait_period(sense_detect_target), msec)
    Sense_Detect -> Sense_Fail [order 1] : [sense_detect_mode == Pace_Sense_Response.Nothing]
    Sense_Detect -> Sense_Fail [order 2] : [after(double(sense_timeout_threshold) - double(sense_wait_period(sense_detect_target)), msec)]
    Sense_Detect -> Sense_Detected [order 3] : [det_sig(sense_detect_target) == true]
  note: SENSE conducts all timing related operations and activates PACE when needed
  SENSE -> PACE : sense_timeout
  PACE -> SENSE : pace_compl
  (default) -> SENSE
  data: p_chamb input Enum: Pace_Chamber; sense_detect_target input; sense_timeout_threshold input; p_pwm input; sense_wait_period input; ATR_PACE_CTRL output; VENT_PACE_CTRL output; PACING_REF_PWM output; PACE_CHARGE_CTRL output; PACE_GND_CTRL output; ATR_GND_CTRL output; VENT_GND_CTRL output; p_width input; sense_detect_mode input Enum: Pace_Sense_Response; det_sig input
  events: sense_timeout local FUNCTION_CALL_EVENT; pace_compl local FUNCTION_CALL_EVENT

== matlab function Assignment1_V6/RATE_SYSTEM/ACCEL_DATA_PREPROCESSOR/ACCEL_SMOOTHER/Buffer Smooth/MATLAB Function ==
  data: input_data input; Buffer_Output output; buffer_length input
function Buffer_Output = Generate_Buffer(input_data, buffer_length)
    persistent Buffer_Internal;
    if (isempty(Buffer_Internal))
        Buffer_Internal = ones(50); %upper bound 1000
    else
        for i = 1:buffer_length-1
            Buffer_Internal(buffer_length-i+1) = Buffer_Internal(buffer_length-i);
        end
        Buffer_Internal(1) = input_data;
    end
    Buffer_Output = Buffer_Internal;
end

== matlab function Assignment1_V6/RATE_SYSTEM/ACCEL_DATA_PREPROCESSOR/ACCEL_SMOOTHER/Buffer Smooth/MATLAB Function1 ==
  data: input_buffer input; Smoothed_Output output; buffer_length input
function Smoothed_Output = Smooth_Output(input_buffer, buffer_length)
    Sum_Value = 0;
    for i = 1:buffer_length
        Sum_Value = Sum_Value + input_buffer(i);
    end
    Smoothed_Output = Sum_Value/buffer_length;
end

== matlab function Assignment1_V6/RATE_SYSTEM/ACCEL_DATA_PREPROCESSOR/CALC_MOTION_STATE/MATLAB Function ==
  data: Input_Activity input; Motion_State output; Input_Activity_Threshold input
function Motion_State = Determine_Motion_State(Input_Activity, Input_Activity_Threshold)
    Motion_State_num = 3;
    for i = 2:-1:1
         if Input_Activity_Threshold(i) > Input_Activity
               Motion_State_num = i;
         end
    end
    Motion_State = Motion_State_num;
end

== stateflow chart Assignment1_V6/Chart ==
  state Save_Buf_Params
    entry:
    Params_Arr = Output_Candidate;
  state Init
    entry:
    Params_Arr = default_params;
    Output_Candidate = default_params;
    %Params_Raw = ones(8,1,'uint8');
    TX_ctrlmode = 2;
  state ECG_TX_Loop_Standby
    entry:
    TX_ctrlmode = 2;
    send_params();
  state Detect_Cur_Mode
    entry:
    Rx_buf = Rx;
    Op_Mode = typecast(Rx_buf(1), 'uint8');
    TX_ctrlmode = 1;
  state Conv_Data
    entry:
    Output_Candidate = Process_Rx(Rx_buf(2:end));
    Rxint_buf = reshape(Rx_buf, 4,4);
    iter = 1;
  state TX_Rxint_buf
    entry:
    Params_Raw = uint8(Rxint_buf(:,iter));
    send_params();
    iter = iter+1;
  state TX_wait
    entry:
  Save_Buf_Params -> ECG_TX_Loop_Standby : [after(20,msec)]
  Detect_Cur_Mode -> Save_Buf_Params [order 2] : [Op_Mode == 255]
  Detect_Cur_Mode -> ECG_TX_Loop_Standby [order 1] : [Op_Mode ~= 255 & Op_Mode ~= 254]
  (default) -> Init
  ECG_TX_Loop_Standby -> ECG_TX_Loop_Standby [order 1] : [after(10,msec)]
  Detect_Cur_Mode -> Conv_Data [order 3] : [Op_Mode == 254]
  Init -> ECG_TX_Loop_Standby
  ECG_TX_Loop_Standby -> Detect_Cur_Mode [order 2] : [Status == 0]
  TX_wait -> ECG_TX_Loop_Standby [order 2] : [after(timeout_threshold, msec)]
  TX_wait -> Detect_Cur_Mode [order 1] : [Status == 0]
  TX_Rxint_buf -> Detect_Cur_Mode [order 2] : [Status == 0]
  Conv_Data -> TX_Rxint_buf : [after(110,msec)]
  TX_Rxint_buf -> TX_Rxint_buf [order 3] : [after(10,msec)]
  TX_Rxint_buf -> TX_wait [order 1] : [iter >= 5]
  data: Rx_input function_input; output_set function_output; Rx input uint8; Status input uint8; Output_Candidate local uint8; Params_Raw output uint8; Op_Mode local uint8; default_params input uint8; timeout_threshold input double; Params_Arr output uint8; TX_ctrlmode output uint8; iter local uint8; Rxint_buf local uint8; Rx_buf local
  events: send_params output FUNCTION_CALL_EVENT
  function output_set = Process_Rx(Rx_input):
    | function output_set = Process_Rx(Rx_input)
    |     output_set = zeros(15,1,'uint8');
    |     for i = 1:15
    |         tmp = typecast(Rx_input(i),'uint8');
    |         output_set(i) = tmp;
    |     end
    | end

== matlab function Assignment1_V6/RATE_SYSTEM/ACCEL_DATA_PREPROCESSOR/ACCEL_SMOOTHER/MATLAB Function2 ==
  data: input input; smoothed_output output; buffer_length input
function smoothed_output = rolling_average_smooth(input, buffer_length)
    persistent rolling_avg;
    persistent init_counter;

    if (isempty(init_counter)) 
        init_counter = 0; 
        rolling_avg = 0;
    end

    if (init_counter < buffer_length)
        init_counter = init_counter + 1;
    end
    rolling_avg = rolling_avg * (init_counter-1)/(init_counter) + input/init_counter;

    smoothed_output = rolling_avg;
end

== stateflow chart Assignment1_V6/RATE_SYSTEM/RATE_CTRL_SYSTEM ==
  state Init
    sense_timeout_threshold = single(p_sense_timeout);
    iter = 0;
  state Pace_LRL_Fixed
    sense_timeout_threshold = single(p_sense_timeout);
  state Detect_Mode
  state Pace_Rate_Unfixed
    state get_tgt
      entry:
      tgt = Calc_Rate_Response(Motion_Magnitude, [2.6, -40],p_sense_timeout, r_sense_timeout_max);
      iter = iter + 1;
      if (iter == 100)
      UPDATE_EXP_FAC();
      iter = 0;
      end
    state Bigger
      sense_timeout_threshold = single((sense_timeout_threshold) + dif * resp_exp_fac(Motion_State + 3));
    state check_dif
      dif = double(tgt - sense_timeout_threshold);
    state Smaller
      sense_timeout_threshold = single((sense_timeout_threshold) + dif * resp_exp_fac(Motion_State));
    (default) -> get_tgt
    (junction 122) -> get_tgt
    get_tgt -> (junction 130) [order 2] : [after(100,msec)]
    (junction 130) -> check_dif : [p_rate_mode ~= Pace_Rate_Mode.Disabled]
    Bigger -> (junction 122)
    Smaller -> (junction 122)
    check_dif -> Bigger [order 1] : [dif >= 0]
    check_dif -> Smaller [order 2] : [dif <= 0]
  get_tgt -> Detect_Mode [order 1] : [p_rate_mode == Pace_Rate_Mode.Disabled]
  (default) -> Init
  Init -> Detect_Mode
  Pace_LRL_Fixed -> Detect_Mode : [p_rate_mode == Pace_Rate_Mode.Enabled]
  Detect_Mode -> Pace_LRL_Fixed [order 1] : [p_rate_mode == Pace_Rate_Mode.Disabled]
  Detect_Mode -> Pace_Rate_Unfixed [order 2] : [p_rate_mode == Pace_Rate_Mode.Enabled]
  data: activity function_input; ratefactors function_input; LRP function_input; MSP function_input; value function_output; Motion_State input; Motion_Magnitude input; r_sense_timeout_max input; p_rate_mode input; sense_timeout_threshold output single size=1; p_sense_timeout input; dif local double; tgt local single; resp_exp_fac input; iter local uint8
  function value = Calc_Rate_Response(activity, ratefactors, LRP, MSP):
    | function value = Calc_Rate_Response(activity, ratefactors, LRP, MSP)
    |     %ratefactors: m, b
    |     value = single(ratefactors(1)*activity + ratefactors(2)); %in bpm
    |     if (value == 0 || value < 0)
    |         value = single(LRP);
    |         return
    |     end
    |     value = 60000/value; %in ms period
    |     if (value > LRP)
    |         value = single(LRP);
    |         return;
    |     end
    |     if (value < MSP)
    |         value = single(MSP);
    |         return;
    |     end
    | end
